simulink library "tether_drag_ul"  (R2018b)
settings: Solver=VariableStepAuto  StartTime=0.0  StopTime=10.0  RelTol=1e-3
settings Model: Creator=Ayaz  LastModifiedBy=Ayaz

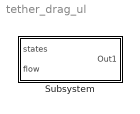
== system tether_drag_ul ==
  Subsystem : Subsystem

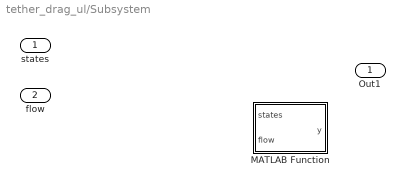
== system tether_drag_ul/Subsystem ==
  states : Inport
  flow : Inport  Port=2
  MATLAB Function : MATLAB Function  TreatAsAtomicUnit=on
  Out1 : Outport

== matlab function tether_drag_ul/Subsystem/MATLAB Function ==
  data: states input; y output; flow input
function y = fcn(states,flow)

X = states;
N = length(states)/6;

Ri_o = X(1:3*N);
Vi_o = X(3*N + 1:6*N);



y = u;
